simulink model "CAN_No_Anomalies"  (R2021a)
settings: Solver=FixedStepDiscrete  StartTime=0.0  StopTime=150  FixedStep=0.005  RelTol=1e-3
undefined symbols (not defined in the file or in its folder): canChannel
libraries: canlib x4, canmsglib x2
settings Model: Creator=saisa  LastModifiedBy=saisa

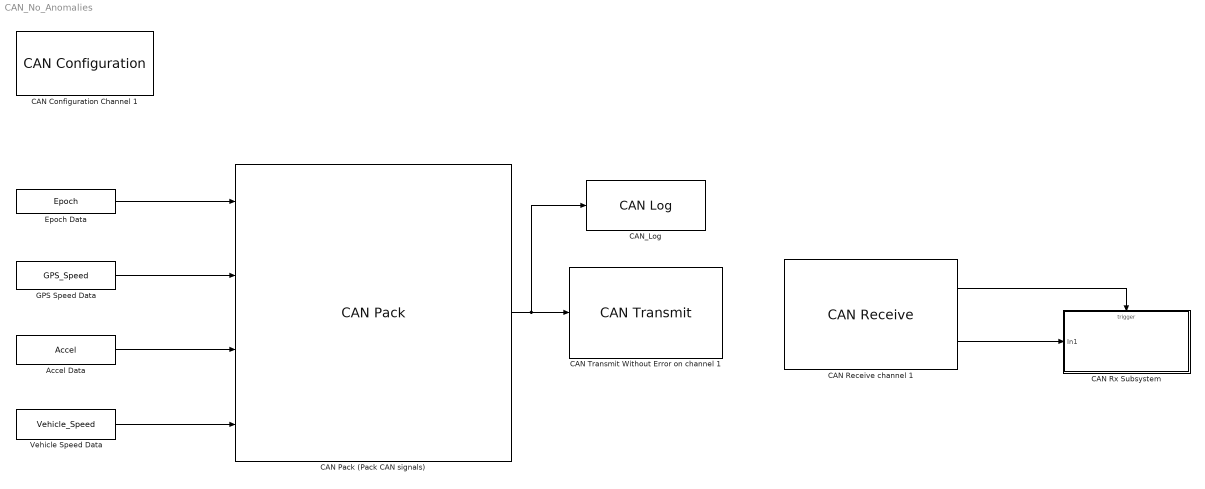
== system CAN_No_Anomalies ==
  Accel Data : FromWorkspace  VariableName=Accel  OutDataTypeStr=double  SampleTime=-1  Interpolate=off  ZeroCross=off  OutputAfterFinalValue=Holding final value
  CAN Configuration Channel 1 : canlib/CAN Configuration  BlockHandle=3.0001  Device=MathWorks Virtual 1 (Channel 1)  DeviceMenu=MathWorks Virtual 1 (Channel 1)  ObjConstructor=canChannel('MathWorks', 'Virtual 1', 1)  BusSpeed=500000  EnableBitParameters=off  AckMode=Normal
      settings: SourceProductBaseCode=VN
  CAN Pack (Pack CAN signals) : canmsglib/CAN Pack  CANdbFile=C:\University\Course_Subjects\Semester_3\Study Project\Implementation\SPMD.dbc  MsgList=WheelSpeeds  MsgName=WheelSpeeds  MsgIDType=Standard (11-bit identifier)  MsgIdentifier=1200  MsgLength=8  Remote=off  ApplyMinMax=off  BusOutput=on  SignalInfo={'Epoch','0','16','LE','unsigned','Standard','0','0.01','0','0','30000';'GPS_Speed','16','16','LE','unsigned','Standard','0','0.01','-100','0','2000';'InVehicle_Longitudinal_Accel','48','16','LE','signed','Standard','0','0.01','-100','-2000','2000';'InVehicle_Longitudinal_Speed','32','16','LE','unsigned','Standard','0','0.01','-100','0','2000'}
      settings: SourceProductBaseCode=ME,XP,VN  DataFormat=CANdb specified signals
  CAN Receive channel 1 : canlib/CAN Receive  BlockHandle=5.0001  Device=MathWorks Virtual 1 (Channel 1)  DeviceMenu=MathWorks Virtual 1 (Channel 1)  ObjConstructor=canChannel('MathWorks', 'Virtual 1', 1)  EnableStandardIDsFilter=off  StdIDsCombo=Allow all  StandardIDs=0  EnableExtendedIDsFilter=off  ExtIDsCombo=Allow all  ExtendedIDs=0  SampleTime=-1  MsgsPerTimestep=all  InternalFilterUpdateStatus=on  BusOutput=off
      settings: SourceProductBaseCode=VN
  CAN Rx Subsystem : Subsystem  TreatAsAtomicUnit=on
  CAN Transmit Without Error on channel 1 : canlib/CAN Transmit  BlockHandle=17.0001  Device=MathWorks Virtual 1 (Channel 1)  DeviceMenu=MathWorks Virtual 1 (Channel 1)  ObjConstructor=canChannel('MathWorks', 'Virtual 1', 1)  EnableEventTransmit=off  EnablePeriodicTransmit=off  MessagePeriod=1.000
      settings: SourceProductBaseCode=VN
  CAN_Log : canlib/CAN Log  BlockHandle=18.0001  FullPathFileName=Without_Error_Tx.mat  FileName=Without_Error_Tx.mat  VariableName=Without_Error_Tx  MaxNumMessages=30000  LogFrom=Input port  DeviceMenu=Select a device  Device=Select a device  ObjConstructor=Select a constructor  SampleTime=0.01
      settings: SourceProductBaseCode=VN
  Epoch Data : FromWorkspace  VariableName=Epoch  OutDataTypeStr=double  SampleTime=-1  Interpolate=off  ZeroCross=off  OutputAfterFinalValue=Holding final value
  GPS Speed Data : FromWorkspace  VariableName=GPS_Speed  OutDataTypeStr=double  SampleTime=-1  Interpolate=off  ZeroCross=off  OutputAfterFinalValue=Holding final value
  Vehicle Speed Data : FromWorkspace  VariableName=Vehicle_Speed  OutDataTypeStr=double  SampleTime=-1  Interpolate=off  ZeroCross=off  OutputAfterFinalValue=Holding final value
  wires:
  CAN Receive channel 1/1 -> CAN Rx Subsystem/Trigger
  CAN Receive channel 1/2 -> CAN Rx Subsystem/1(In1)
  Accel Data/1 -> CAN Pack (Pack CAN signals)/3
  GPS Speed Data/1 -> CAN Pack (Pack CAN signals)/2
  Epoch Data/1 -> CAN Pack (Pack CAN signals)/1
  Vehicle Speed Data/1 -> CAN Pack (Pack CAN signals)/4
  CAN Pack (Pack CAN signals)/1 -> CAN_Log/1, CAN Transmit Without Error on channel 1/1

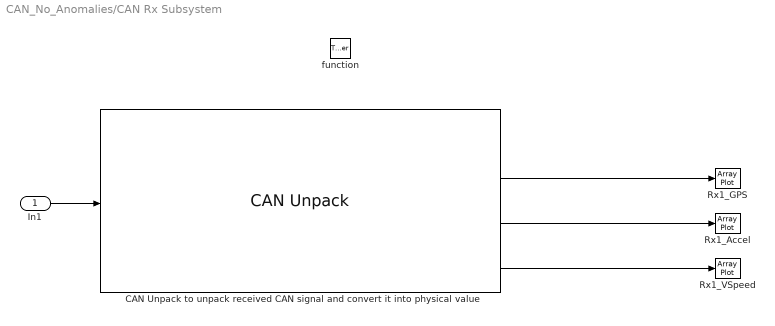
== system CAN_No_Anomalies/CAN Rx Subsystem ==
  In1 : Inport
  function : TriggerPort  TriggerType=function-call  VariantControl=(inherit)
  CAN Unpack to unpack received CAN signal and convert it into physical value : canmsglib/CAN Unpack  CANdbFile=C:\University\Course_Subjects\Semester_3\Study Project\Implementation\SPMD.dbc  MsgList=WheelSpeeds  MsgName=WheelSpeeds  MsgIDType=Standard (11-bit identifier)  MsgIdentifier=1200  MsgLength=8  SignalInfo={'Epoch','0','16','LE','unsigned','Standard','0','0.01','0','0','30000';'GPS_Speed','16','16','LE','unsigned','Standard','0','0.01','-100','0','2000';'InVehicle_Longitudinal_Accel','48','16','LE','signed','Standard','0','0.01','-100','-2000','2000';'InVehicle_Longitudinal_Speed','32','16','LE','unsigned','Standard','0','0.01','-100','0','2000'}  IDPort=off  TimestampPort=off  ErrorPort=off  RemotePort=off  LengthPort=off  StatusPort=off  ApplyMinMax=off
      settings: SourceProductBaseCode=ME,XP,VN  DataFormat=CANdb specified signals
  Rx1_Accel : ArrayPlot  WindowPosition=[240.000000,110.000000,800.000000,500.000000,]  Visible=on  DefaultConfigurationName=dsp.scopes.ArrayPlotBlockSpecification
  Rx1_GPS : ArrayPlot  WindowPosition=[240.000000,110.000000,800.000000,500.000000,]  Visible=on  DefaultConfigurationName=dsp.scopes.ArrayPlotBlockSpecification
  Rx1_VSpeed : ArrayPlot  WindowPosition=[240.000000,110.000000,800.000000,500.000000,]  Visible=on  DefaultConfigurationName=dsp.scopes.ArrayPlotBlockSpecification
  wires:
  In1/1 -> CAN Unpack to unpack received CAN signal and convert it into physical value/1
  CAN Unpack to unpack received CAN signal and convert it into physical value/4 -> Rx1_VSpeed/1
  CAN Unpack to unpack received CAN signal and convert it into physical value/3 -> Rx1_Accel/1
  CAN Unpack to unpack received CAN signal and convert it into physical value/2 -> Rx1_GPS/1
